simulink model "FullSystem_threshold_fix_attempt"  (R2014a)
settings: Solver=FixedStepDiscrete  StartTime=0.0  StopTime=1.5  FixedStep=1/8000  RelTol=1e-3
undefined symbols (not defined in the file): i
libraries: dspmtrx3 x7, dspsrcs4 x7, commutil2 x1, dspstat3 x1, dspsigops x1, dspbuff3 x1, simulink x1
settings Model: NumberOfSteps=400  Creator=Dolby  LastModifiedBy=100442260
settings DataIOCC: SaveOutput=off  SaveTime=off
settings DebuggingCC: UnderspecifiedInitializationDetection=Classic  StateNameClashWarn=warning

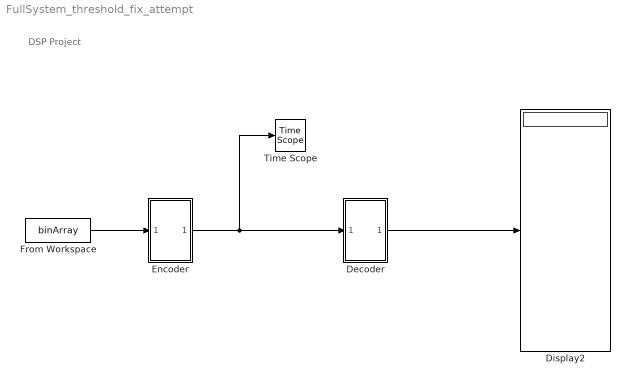
== system FullSystem_threshold_fix_attempt ==
  note: DSP Project
  "Decoder " : Subsystem
  Display2 : Display
  Encoder : Subsystem
  From Workspace : FromWorkspace  VariableName=binArray
  Time Scope : TimeScope  DefaultConfigurationName=spbscopes.TimeScopeBlockCfg
  wires:
  Encoder/1(Out1) -> "Decoder "/1(In1), Time Scope/1
  From Workspace/1 -> Encoder/1(In1)
  "Decoder "/1(Out1) -> Display2/1

== system FullSystem_threshold_fix_attempt/Decoder  ==
  In1 : Inport
  Binary to Decimal : Subsystem
  Delay : Delay  DelayLength=60  InitialCondition=0
  Digitbreak : Subsystem
  "Geortzel Filtering " : Subsystem
  Shift register : Subsystem  TreatAsAtomicUnit=on
  Time Scope1 : TimeScope  DefaultConfigurationName=spbscopes.TimeScopeBlockCfg
  Out1 : Outport
  wires:
  In1/1 -> Digitbreak/1(In1), "Geortzel Filtering "/1(In1)
  "Geortzel Filtering "/1(Out1) -> Binary to Decimal/1(In1)
  Shift register/1(Output) -> Out1/1
  Digitbreak/1(Out2) -> Time Scope1/1, Delay/1, Binary to Decimal/2(In2), "Geortzel Filtering "/2(In2)  "Trigger"
  Binary to Decimal/1(Out2) -> Shift register/1(Input)
  Delay/1 -> Shift register/Trigger

== system FullSystem_threshold_fix_attempt/Encoder ==
  In1 : Inport
  Noise : Subsystem
  Tone Generator : Subsystem
  Out1 : Outport
  wires:
  In1/1 -> Tone Generator/1(In1)
  Tone Generator/1(Out1) -> Noise/1(In1)
  Noise/1(Out1) -> Out1/1

== system FullSystem_threshold_fix_attempt/Decoder /Binary to Decimal ==
  In1 : Inport
  In2 : Inport  Port=2
  Delay : Delay  DelayLength=60  InitialCondition=0
  Triggered Subsystem : Subsystem  TreatAsAtomicUnit=on
  Out2 : Outport
  wires:
  Delay/1 -> Triggered Subsystem/Trigger
  In1/1 -> Triggered Subsystem/1(In1)
  In2/1 -> Delay/1
  Triggered Subsystem/1(Out1) -> Out2/1

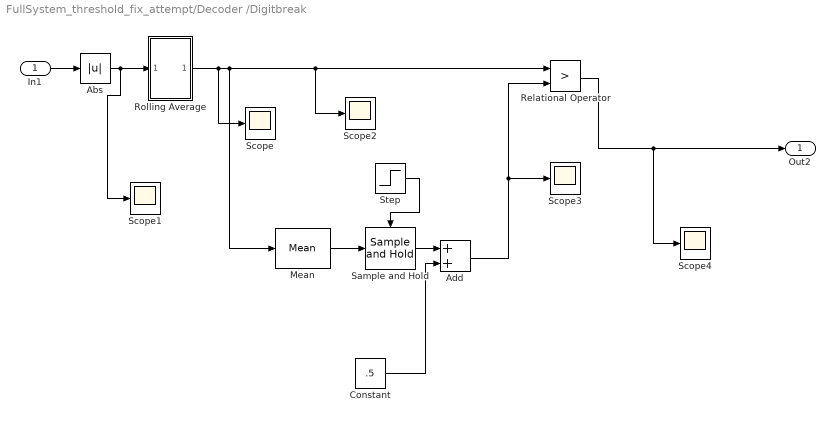
== system FullSystem_threshold_fix_attempt/Decoder /Digitbreak ==
  In1 : Inport
  Abs : Abs
  Add : Sum
  Constant : Constant  Value=.5
  Mean : dspstat3/Mean  run=on  reset_popup=None  InputProcessing=Columns as channels (frame based)  directionMode=Each column  dimension=1  treatSBRowAsCol=on  roiEnable=off  roiType=Rectangles  roiPortion=Entire ROI  roiOutput=Individual statistics for each ROI  roiFlag=off  outputDataTypeStr=Inherit: Same as accumulator  outputLastDataTypeStr=Inherit: Same as accumulator  outputMin=[]  outputMax=[]  roundingMode=Floor  overflowMode=off
  Relational Operator : RelationalOperator  Operator=>  OutDataTypeStr=boolean
  Rolling Average : Subsystem
  Sample and Hold : dspsigops/Sample and Hold  trig=Rising edge  initCond=.5  latchinput=off
  Scope{,1..4} (5 alike) : Scope
      Scope settings: SaveName=ScopeData21
      Scope1 settings: SaveName=ScopeData19
      Scope2 settings: SaveName=ScopeData20
      Scope3 settings: SaveName=ScopeData7
      Scope4 settings: SaveName=ScopeData24
  Step : Step  Time=.05  SampleTime=0
  Out2 : Outport
  wires:
  Abs/1 -> Scope1/1, Rolling Average/1(In1)
  In1/1 -> Abs/1
  Relational Operator/1 -> Scope4/1, Out2/1
  Step/1 -> Sample and Hold/Trigger
  Rolling Average/1(Out1) -> Scope/1, Scope2/1, Relational Operator/1, Mean/1
  Mean/1 -> Sample and Hold/1
  Add/1 -> Scope3/1, Relational Operator/2
  Sample and Hold/1 -> Add/1
  Constant/1 -> Add/2

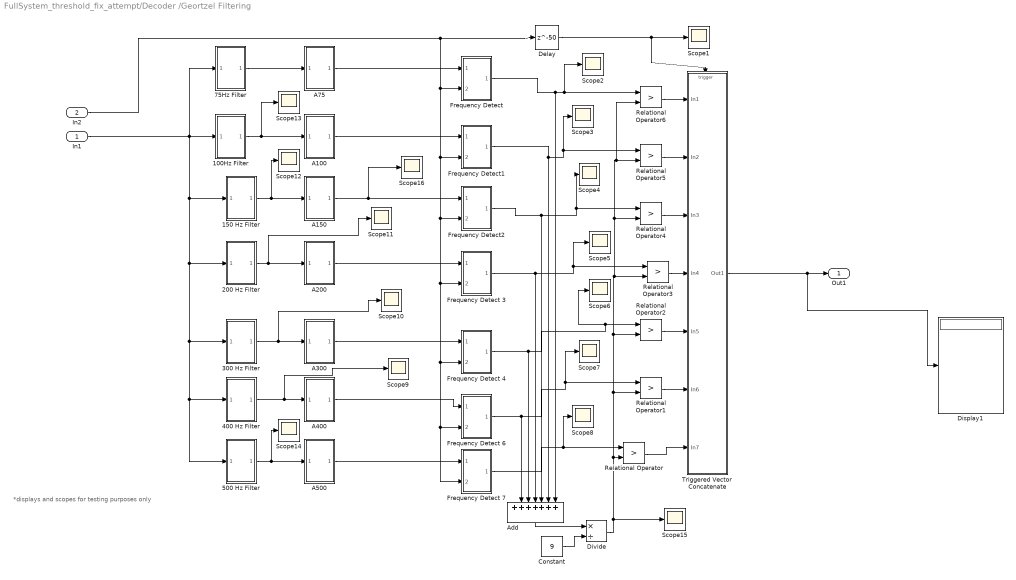
== system FullSystem_threshold_fix_attempt/Decoder /Geortzel Filtering  ==
  note: *displays and scopes for testing purposes only
  In1 : Inport
  In2 : Inport  Port=2
  100Hz Filter : Subsystem
  150 Hz Filter : Subsystem
  200 Hz Filter : Subsystem
  "300 Hz Filter " : Subsystem
  400 Hz Filter : Subsystem
  500 Hz Filter : Subsystem
  75Hz Filter : Subsystem
  A100 : Subsystem
  A150 : Subsystem
  "A200 " : Subsystem
  A300 : Subsystem
  A400 : Subsystem
  A500 : Subsystem
  A75 : Subsystem
  Add : Sum  Inputs=+++++++
  Constant : Constant  Value=9
  Delay : Delay  DelayLength=50  InitialCondition=0
  Display1 : Display
  Divide : Product  Inputs=*/
  Frequency Detect : Subsystem
  "Frequency Detect 3 " : Subsystem
  Frequency Detect 4 : Subsystem
  "Frequency Detect 6 " : Subsystem
  "Frequency Detect 7 " : Subsystem
  "Frequency Detect1 " : Subsystem
  "Frequency Detect2 " : Subsystem
  Relational Operator{,1..6} (7 alike) : RelationalOperator  Operator=>  OutDataTypeStr=boolean
  Scope{1..16} (16 alike) : Scope
      Scope1 settings: TimeRange=0.2  YMin=-2  YMax=2
      Scope10 settings: TimeRange=0.2  YMin=-2  YMax=2  SaveName=ScopeData12
      Scope11 settings: TimeRange=0.2  YMin=-2  YMax=2  SaveName=ScopeData13
      Scope12 settings: TimeRange=0.2  YMin=-2  YMax=2  SaveName=ScopeData14
      Scope13 settings: TimeRange=0.2  YMin=-2  YMax=2  SaveName=ScopeData15
      Scope14 settings: TimeRange=0.2  YMin=-2  YMax=2  SaveName=ScopeData16
      Scope15 settings: TimeRange=0.08000000000000002  YMin=-0.1  YMax=1.3
      Scope16 settings: TimeRange=0.2  YMin=-2  YMax=2  SaveName=ScopeData17
      Scope2 settings: TimeRange=0.2  YMin=-2  YMax=2  SaveName=ScopeData2
      Scope3 settings: TimeRange=0.2  YMin=-2  YMax=2  SaveName=ScopeData4
      Scope4 settings: TimeRange=0.2  YMin=-2  YMax=2  SaveName=ScopeData5
      Scope5 settings: TimeRange=0.2  YMin=-2  YMax=2  SaveName=ScopeData6
      Scope6 settings: TimeRange=0.2  YMin=-2  YMax=2  SaveName=ScopeData8
      Scope7 settings: TimeRange=0.2  YMin=-2  YMax=2  SaveName=ScopeData9
      Scope8 settings: TimeRange=0.2  YMin=-2  YMax=2  SaveName=ScopeData10
      Scope9 settings: TimeRange=0.2  YMin=-2  YMax=2  SaveName=ScopeData11
  Triggered Vector Concatenate : Subsystem
  Out1 : Outport
  wires:
  100Hz Filter/1(Out1) -> Scope13/1, A100/1(In1)
  "300 Hz Filter "/1(Out1) -> Scope10/1, A300/1(In1)
  75Hz Filter/1(Out1) -> A75/1(In1)
  150 Hz Filter/1(Out1) -> Scope12/1, A150/1(In1)
  500 Hz Filter/1(Out1) -> Scope14/1, A500/1(In1)
  A75/1(Out1) -> Frequency Detect/1(In3)
  In1/1 -> 400 Hz Filter/1(In1), 500 Hz Filter/1(In1), "300 Hz Filter "/1(In1), 200 Hz Filter/1(In1), 150 Hz Filter/1(In1), 75Hz Filter/1(In1), 100Hz Filter/1(In1)
  A100/1(Out1) -> "Frequency Detect1 "/1(In3)
  In2/1 -> Frequency Detect/2(In1), "Frequency Detect 7 "/2(In1), "Frequency Detect 6 "/2(In1), Frequency Detect 4/2(In1), "Frequency Detect 3 "/2(In1), "Frequency Detect2 "/2(In1), "Frequency Detect1 "/2(In1), Delay/1
  A150/1(Out1) -> Scope16/1, "Frequency Detect2 "/1(In3)
  "A200 "/1(Out1) -> "Frequency Detect 3 "/1(In3)
  A300/1(Out1) -> Frequency Detect 4/1(In3)
  A400/1(Out1) -> "Frequency Detect 6 "/1(In3)
  A500/1(Out1) -> "Frequency Detect 7 "/1(In3)
  "Frequency Detect2 "/1(Out1) -> Scope4/1, Relational Operator4/1, Add/5
  "Frequency Detect 3 "/1(Out1) -> Add/4, Relational Operator3/1, Scope5/1
  Frequency Detect 4/1(Out1) -> Add/3, Relational Operator2/1, Scope6/1
  "Frequency Detect 6 "/1(Out1) -> Add/2, Relational Operator1/1, Scope7/1
  "Frequency Detect 7 "/1(Out1) -> Relational Operator/1, Scope8/1
  Delay/1 -> Scope1/1, Triggered Vector Concatenate/Trigger
  Triggered Vector Concatenate/1(Out1) -> Out1/1, Display1/1
  200 Hz Filter/1(Out1) -> Scope11/1, "A200 "/1(In1)
  400 Hz Filter/1(Out1) -> Scope9/1, A400/1(In1)
  Relational Operator/1 -> Triggered Vector Concatenate/7(In7)
  Add/1 -> Divide/1
  Constant/1 -> Divide/2
  Relational Operator1/1 -> Triggered Vector Concatenate/6(In6)
  Relational Operator2/1 -> Triggered Vector Concatenate/5(In5)
  Divide/1 -> Scope15/1, Relational Operator6/2, Relational Operator5/2, Relational Operator4/2, Relational Operator3/2, Relational Operator2/2, Relational Operator1/2, Relational Operator/2
  Relational Operator3/1 -> Triggered Vector Concatenate/4(In4)
  Relational Operator4/1 -> Triggered Vector Concatenate/3(In3)
  Relational Operator5/1 -> Triggered Vector Concatenate/2(In2)
  Relational Operator6/1 -> Triggered Vector Concatenate/1(In1)
  Frequency Detect/1(Out1) -> Add/7, Relational Operator6/1, Scope2/1
  "Frequency Detect1 "/1(Out1) -> Add/6, Relational Operator5/1, Scope3/1

== system FullSystem_threshold_fix_attempt/Decoder /Shift register ==
  Input : Inport
  Trigger : TriggerPort  TriggerType=falling  ZeroCross=off
  Delay Line : dspbuff3/Delay Line  siz=11  ic=0  directfeed=on  enable_output=off  hold_output=off  TreatMby1Signals=One channel
  Output : Outport
  wires:
  Input/1 -> Delay Line/1
  Delay Line/1 -> Output/1

== system FullSystem_threshold_fix_attempt/Encoder/Noise ==
  In1 : Inport
  Add : Sum
  Band-Limited White Noise : simulink/Sources/Band-Limited White Noise  Cov=[0.0000005]  Ts=1/8000  seed=[1]
  Scope : Scope
      settings: SaveName=ScopeData22
  Out1 : Outport
  wires:
  In1/1 -> Add/2
  Band-Limited White Noise/1 -> Add/1
  Add/1 -> Scope/1, Out1/1

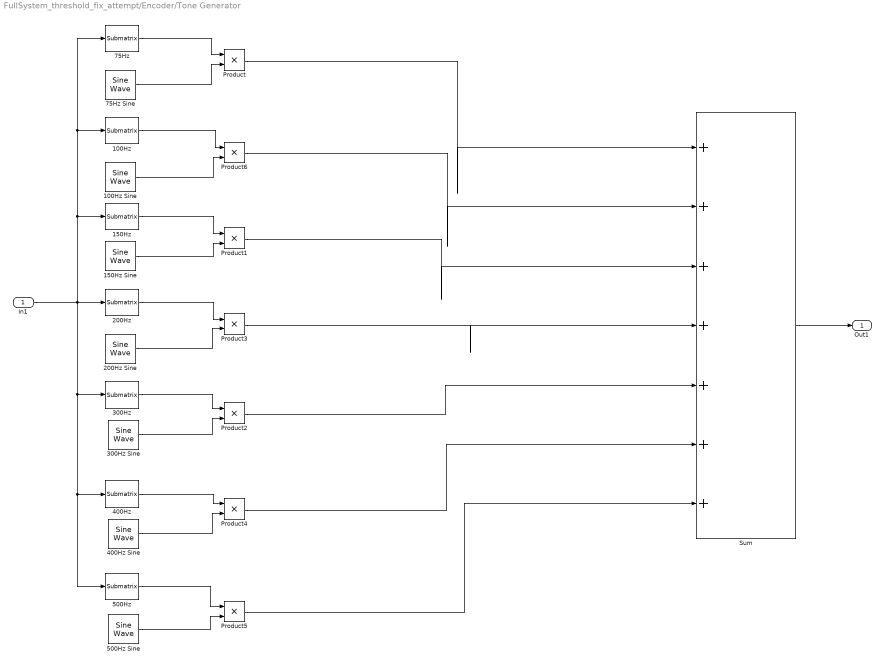
== system FullSystem_threshold_fix_attempt/Encoder/Tone Generator ==
  In1 : Inport
  100Hz : dspmtrx3/Submatrix  RowSpan=One row  RowStartMode=Index  RowStartIndex=2  RowEndMode=Last  RowEndIndex=1  ColSpan=Range of columns  ColStartMode=First  ColStartIndex=1  ColEndMode=Last  ColEndIndex=1
  100Hz Sine : dspsrcs4/Sine Wave  Amplitude=1 + rand()  Frequency=100  Phase=0  SampleMode=Discrete  OutComplex=Real  CompMethod=Trigonometric fcn  TableSize=Speed  SampleTime=1/8000  SamplesPerFrame=1  ResetState=Restart at time zero  dataType=double  wordLen=16  udDataType=sfix(16)  fracBitsMode=Best precision  numFracBits=15  OutDataTypeStr=double  LastOutDataTypeStr=double
  150Hz : dspmtrx3/Submatrix  RowSpan=One row  RowStartMode=Index  RowStartIndex=3  RowEndMode=Last  RowEndIndex=1  ColSpan=Range of columns  ColStartMode=First  ColStartIndex=1  ColEndMode=Last  ColEndIndex=1
  150Hz Sine : dspsrcs4/Sine Wave  Amplitude=1 + rand()  Frequency=150  Phase=0  SampleMode=Discrete  OutComplex=Real  CompMethod=Trigonometric fcn  TableSize=Speed  SampleTime=1/8000  SamplesPerFrame=1  ResetState=Restart at time zero  dataType=double  wordLen=16  udDataType=sfix(16)  fracBitsMode=Best precision  numFracBits=15  OutDataTypeStr=double  LastOutDataTypeStr=double
  200Hz : dspmtrx3/Submatrix  RowSpan=One row  RowStartMode=Index  RowStartIndex=4  RowEndMode=Last  RowEndIndex=1  ColSpan=Range of columns  ColStartMode=First  ColStartIndex=1  ColEndMode=Last  ColEndIndex=1
  200Hz Sine : dspsrcs4/Sine Wave  Amplitude=1 + rand()  Frequency=200  Phase=0  SampleMode=Discrete  OutComplex=Real  CompMethod=Trigonometric fcn  TableSize=Speed  SampleTime=1/8000  SamplesPerFrame=1  ResetState=Restart at time zero  dataType=double  wordLen=16  udDataType=sfix(16)  fracBitsMode=Best precision  numFracBits=15  OutDataTypeStr=double  LastOutDataTypeStr=double
  300Hz : dspmtrx3/Submatrix  RowSpan=One row  RowStartMode=Index  RowStartIndex=5  RowEndMode=Last  RowEndIndex=1  ColSpan=Range of columns  ColStartMode=First  ColStartIndex=1  ColEndMode=Last  ColEndIndex=1
  300Hz Sine : dspsrcs4/Sine Wave  Amplitude=1 + rand()  Frequency=300  Phase=0  SampleMode=Discrete  OutComplex=Real  CompMethod=Trigonometric fcn  TableSize=Speed  SampleTime=1/8000  SamplesPerFrame=1  ResetState=Restart at time zero  dataType=double  wordLen=16  udDataType=sfix(16)  fracBitsMode=Best precision  numFracBits=15  OutDataTypeStr=double  LastOutDataTypeStr=double
  400Hz : dspmtrx3/Submatrix  RowSpan=One row  RowStartMode=Index  RowStartIndex=6  RowEndMode=Last  RowEndIndex=1  ColSpan=Range of columns  ColStartMode=First  ColStartIndex=1  ColEndMode=Last  ColEndIndex=1
  400Hz Sine : dspsrcs4/Sine Wave  Amplitude=1 + rand()  Frequency=400  Phase=0  SampleMode=Discrete  OutComplex=Real  CompMethod=Trigonometric fcn  TableSize=Speed  SampleTime=1/8000  SamplesPerFrame=1  ResetState=Restart at time zero  dataType=double  wordLen=16  udDataType=sfix(16)  fracBitsMode=Best precision  numFracBits=15  OutDataTypeStr=double  LastOutDataTypeStr=double
  500Hz : dspmtrx3/Submatrix  RowSpan=One row  RowStartMode=Last  RowStartIndex=1  RowEndMode=Last  RowEndIndex=1  ColSpan=Range of columns  ColStartMode=First  ColStartIndex=1  ColEndMode=Last  ColEndIndex=1
  500Hz Sine : dspsrcs4/Sine Wave  Amplitude=1 + rand()  Frequency=500  Phase=0  SampleMode=Discrete  OutComplex=Real  CompMethod=Trigonometric fcn  TableSize=Speed  SampleTime=1/8000  SamplesPerFrame=1  ResetState=Restart at time zero  dataType=double  wordLen=16  udDataType=sfix(16)  fracBitsMode=Best precision  numFracBits=15  OutDataTypeStr=double  LastOutDataTypeStr=double
  75Hz : dspmtrx3/Submatrix  RowSpan=One row  RowStartMode=First  RowStartIndex=1  RowEndMode=Last  RowEndIndex=1  ColSpan=Range of columns  ColStartMode=First  ColStartIndex=1  ColEndMode=Last  ColEndIndex=1
  75Hz Sine : dspsrcs4/Sine Wave  Amplitude=1 + rand()  Frequency=75  Phase=0  SampleMode=Discrete  OutComplex=Real  CompMethod=Trigonometric fcn  TableSize=Speed  SampleTime=1/8000  SamplesPerFrame=1  ResetState=Restart at time zero  dataType=double  wordLen=16  udDataType=sfix(16)  fracBitsMode=Best precision  numFracBits=15  OutDataTypeStr=double  LastOutDataTypeStr=double
  Product{,1..6} (7 alike) : Product
  Sum : Sum  Inputs=|+++++++
  Out1 : Outport
  wires:
  150Hz/1 -> Product1/1
  150Hz Sine/1 -> Product1/2
  200Hz/1 -> Product3/1
  100Hz Sine/1 -> Product6/2
  100Hz/1 -> Product6/1
  300Hz/1 -> Product2/1
  75Hz/1 -> Product/1
  400Hz/1 -> Product4/1
  500Hz/1 -> Product5/1
  Product/1 -> Sum/1
  Product6/1 -> Sum/2
  Product1/1 -> Sum/3
  Product3/1 -> Sum/4
  Product2/1 -> Sum/5
  Product4/1 -> Sum/6
  Product5/1 -> Sum/7
  Sum/1 -> Out1/1
  75Hz Sine/1 -> Product/2
  200Hz Sine/1 -> Product3/2
  300Hz Sine/1 -> Product2/2
  400Hz Sine/1 -> Product4/2
  500Hz Sine/1 -> Product5/2
  In1/1 -> 200Hz/1, 150Hz/1, 100Hz/1, 75Hz/1, 300Hz/1, 400Hz/1, 500Hz/1

== system FullSystem_threshold_fix_attempt/Decoder /Binary to Decimal/Triggered Subsystem ==
  In1 : Inport
  Trigger : TriggerPort  TriggerType=falling
  A1 : Constant  Value=[0; 1; 2; 3; 4; 5; 6; 7; 8; 9]
  A11 : Constant  Value=[84; 44; 42; 41; 52; 50; 49; 76; 74; 73]
  Bit to Integer Converter : commutil2/Bit to Integer Converter  nbits=7  bitOrder=MSB first  signedOutputValues=Unsigned  outDtype=Inherit via internal rule  outDtypeSigned=Inherit via internal rule
  Display : Display
  Matrix Sum : Sum  Inputs=+  OutDataTypeStr=double
  Matrix Multiply : Product
  Relational Operator : RelationalOperator  Operator===  OutDataTypeStr=boolean
  Out1 : Outport
  wires:
  A11/1 -> Relational Operator/2
  Matrix Sum/1 -> Out1/1
  In1/1 -> Bit to Integer Converter/1
  Bit to Integer Converter/1 -> Display/1, Relational Operator/1
  Relational Operator/1 -> Matrix Multiply/1
  A1/1 -> Matrix Multiply/2
  Matrix Multiply/1 -> Matrix Sum/1

== system FullSystem_threshold_fix_attempt/Decoder /Digitbreak/Rolling Average ==
  In1 : Inport
  Subsystem : Subsystem
  Out1 : Outport
  wires:
  In1/1 -> Subsystem/1(In1)
  Subsystem/1(Out1) -> Out1/1

== system FullSystem_threshold_fix_attempt/Decoder /Geortzel Filtering /100Hz Filter ==
  In1 : Inport
  Add3 : Sum
  Add4 : Sum  Inputs=-+
  Add5 : Sum
  Gain3 : Gain
  Gain4 : Gain  Gain=-cos(2*pi*5/400)-(sin(2*pi*5/400)*i)
  Gain5 : Gain  Gain=2*cos(2*pi*5/400)
  Unit Delay : UnitDelay  SampleTime=-1
  Unit Delay1 : UnitDelay  SampleTime=-1
  Out1 : Outport
  wires:
  In1/1 -> Add3/1
  Add4/1 -> Add3/2
  Gain3/1 -> Add4/1
  Add3/1 -> Unit Delay/1, Add5/1
  Add5/1 -> Out1/1
  Gain5/1 -> Add4/2
  Gain4/1 -> Add5/2
  Unit Delay1/1 -> Gain3/1
  Unit Delay/1 -> Gain4/1, Unit Delay1/1, Gain5/1

== system FullSystem_threshold_fix_attempt/Decoder /Geortzel Filtering /150 Hz Filter ==
  In1 : Inport
  Add6 : Sum
  Add7 : Sum  Inputs=-+
  Add8 : Sum
  Gain6 : Gain
  Gain7 : Gain  Gain=-cos(2*pi*7.5/400)-(sin(2*pi*7.5/400)*i)
  Gain8 : Gain  Gain=2*cos(2*pi*7.5/400)
  Unit Delay : UnitDelay  SampleTime=-1
  Unit Delay1 : UnitDelay  SampleTime=-1
  Out1 : Outport
  wires:
  In1/1 -> Add6/1
  Gain7/1 -> Add8/2
  Add8/1 -> Out1/1
  Gain8/1 -> Add7/2
  Add7/1 -> Add6/2
  Gain6/1 -> Add7/1
  Add6/1 -> Unit Delay/1, Add8/1
  Unit Delay1/1 -> Gain6/1
  Unit Delay/1 -> Gain7/1, Unit Delay1/1, Gain8/1

== system FullSystem_threshold_fix_attempt/Decoder /Geortzel Filtering /200 Hz Filter ==
  In1 : Inport
  Add10 : Sum  Inputs=-+
  Add11 : Sum
  Add9 : Sum
  Gain10 : Gain  Gain=-cos(2*pi*10/400)-(sin(2*pi*10/400)*i)
  Gain11 : Gain  Gain=2*cos(2*pi*10/400)
  Gain9 : Gain
  Unit Delay : UnitDelay  SampleTime=-1
  Unit Delay1 : UnitDelay  SampleTime=-1
  Out1 : Outport
  wires:
  Gain10/1 -> Add11/2
  Unit Delay1/1 -> Unit Delay/1, Gain10/1, Gain11/1
  Gain9/1 -> Add10/1
  Add10/1 -> Add9/2
  Unit Delay/1 -> Gain9/1
  Add11/1 -> Out1/1
  Add9/1 -> Unit Delay1/1, Add11/1
  Gain11/1 -> Add10/2
  In1/1 -> Add9/1

== system FullSystem_threshold_fix_attempt/Decoder /Geortzel Filtering /300 Hz Filter  ==
  In1 : Inport
  Add12 : Sum
  Add13 : Sum  Inputs=-+
  Add14 : Sum
  Gain12 : Gain
  Gain13 : Gain  Gain=-cos(2*pi*15/400)-(sin(2*pi*15/400)*i)
  Gain14 : Gain  Gain=2*cos(2*pi*15/400)
  Unit Delay : UnitDelay  SampleTime=-1
  Unit Delay1 : UnitDelay  SampleTime=-1
  Out1 : Outport
  wires:
  Add14/1 -> Out1/1
  Add12/1 -> Unit Delay1/1, Add14/1
  Gain12/1 -> Add13/1
  Unit Delay1/1 -> Unit Delay/1, Gain13/1, Gain14/1
  Add13/1 -> Add12/2
  Gain13/1 -> Add14/2
  Unit Delay/1 -> Gain12/1
  Gain14/1 -> Add13/2
  In1/1 -> Add12/1

== system FullSystem_threshold_fix_attempt/Decoder /Geortzel Filtering /400 Hz Filter ==
  In1 : Inport
  Add18 : Sum
  Add19 : Sum  Inputs=-+
  Add20 : Sum
  Gain18 : Gain
  Gain19 : Gain  Gain=-cos(2*pi*21/400)-(sin(2*pi*20/400)*i)  SampleTime=1/8000
  Gain20 : Gain  Gain=2*cos(2*pi*20/400)  SampleTime=1/8000
  Unit Delay : UnitDelay  SampleTime=-1
  Unit Delay1 : UnitDelay  SampleTime=-1
  Out1 : Outport
  wires:
  Unit Delay1/1 -> Unit Delay/1, Gain19/1, Gain20/1
  Add19/1 -> Add18/2
  Add18/1 -> Unit Delay1/1, Add20/1
  Gain18/1 -> Add19/1
  Unit Delay/1 -> Gain18/1
  Add20/1 -> Out1/1
  Gain19/1 -> Add20/2
  Gain20/1 -> Add19/2
  In1/1 -> Add18/1

== system FullSystem_threshold_fix_attempt/Decoder /Geortzel Filtering /500 Hz Filter ==
  In1 : Inport
  Add18 : Sum
  Add19 : Sum  Inputs=-+
  Add20 : Sum
  Gain18 : Gain
  Gain19 : Gain  Gain=-cos(2*pi*25/400)-(sin(2*pi*25/400)*i)
  Gain20 : Gain  Gain=2*cos(2*pi*25/400)
  Unit Delay : UnitDelay  SampleTime=-1
  Unit Delay1 : UnitDelay  SampleTime=-1
  Out1 : Outport
  wires:
  Unit Delay1/1 -> Unit Delay/1, Gain19/1, Gain20/1
  Add19/1 -> Add18/2
  Add18/1 -> Unit Delay1/1, Add20/1
  Gain18/1 -> Add19/1
  Unit Delay/1 -> Gain18/1
  Add20/1 -> Out1/1
  Gain19/1 -> Add20/2
  Gain20/1 -> Add19/2
  In1/1 -> Add18/1

== system FullSystem_threshold_fix_attempt/Decoder /Geortzel Filtering /75Hz Filter ==
  In1 : Inport
  Add : Sum  InputSameDT=on
  Add1 : Sum  Inputs=-+
  Add2 : Sum  InputSameDT=on
  Gain : Gain
  Gain1 : Gain  Gain=-cos(2*pi*3.75/400)-(sin(2*pi*3.75/400)*i)
  Gain2 : Gain  Gain=2*cos(2*pi*3.75/400)
  Unit Delay : UnitDelay  SampleTime=-1
  Unit Delay1 : UnitDelay  SampleTime=-1
  Out1 : Outport
  wires:
  In1/1 -> Add/1
  Add2/1 -> Out1/1
  Gain/1 -> Add1/1
  Gain2/1 -> Add1/2
  Gain1/1 -> Add2/2
  Add1/1 -> Add/2
  Add/1 -> Unit Delay/1, Add2/1
  Unit Delay1/1 -> Gain/1
  Unit Delay/1 -> Unit Delay1/1, Gain1/1, Gain2/1

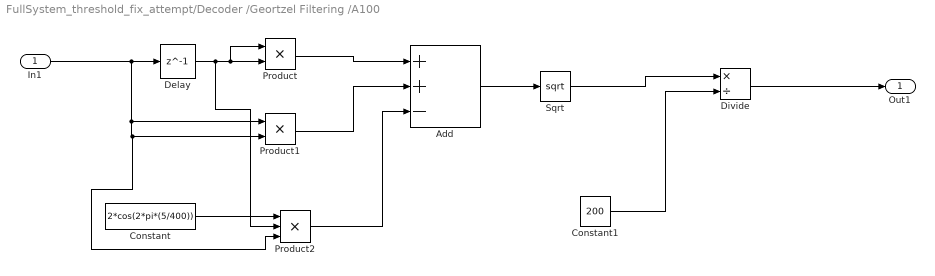
== system FullSystem_threshold_fix_attempt/Decoder /Geortzel Filtering /A100 ==
  In1 : Inport
  Add : Sum  Inputs=++-
  Constant : Constant  Value=2*cos(2*pi*(5/400))
  Constant1 : Constant  Value=200
  Delay : Delay  DelayLength=1  InitialCondition=0
  Divide : Product  Inputs=*/
  Product : Product
  Product1 : Product
  Product2 : Product  Inputs=3
  Sqrt : Sqrt  SaturateOnIntegerOverflow=on
  Out1 : Outport
  wires:
  In1/1 -> Delay/1, Product2/3, Product1/2, Product1/1
  Delay/1 -> Product2/2, Product/1, Product/2
  Product/1 -> Add/1
  Product1/1 -> Add/2
  Constant/1 -> Product2/1
  Add/1 -> Sqrt/1
  Product2/1 -> Add/3
  Sqrt/1 -> Divide/1
  Constant1/1 -> Divide/2
  Divide/1 -> Out1/1

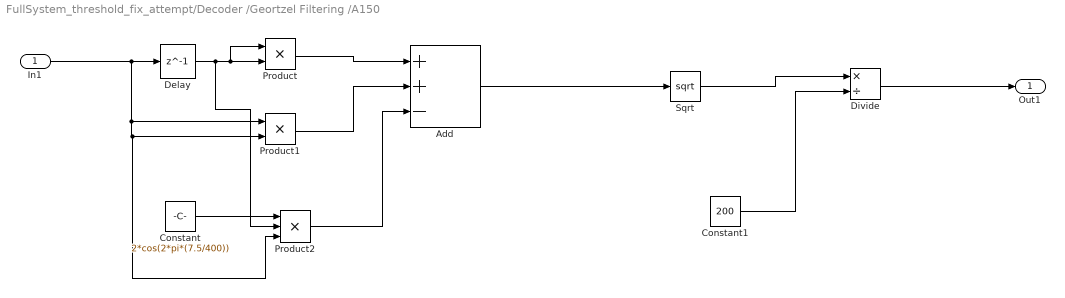
== system FullSystem_threshold_fix_attempt/Decoder /Geortzel Filtering /A150 ==
  In1 : Inport
  Add : Sum  Inputs=++-
  Constant : Constant  Value=2*cos(2*pi*(7.5/400))
  Constant1 : Constant  Value=200
  Delay : Delay  DelayLength=1  InitialCondition=0
  Divide : Product  Inputs=*/
  Product : Product
  Product1 : Product
  Product2 : Product  Inputs=3
  Sqrt : Sqrt  SaturateOnIntegerOverflow=on
  Out1 : Outport
  wires:
  In1/1 -> Delay/1, Product2/3, Product1/2, Product1/1
  Delay/1 -> Product2/2, Product/1, Product/2
  Product/1 -> Add/1
  Product1/1 -> Add/2
  Constant/1 -> Product2/1
  Add/1 -> Sqrt/1
  Product2/1 -> Add/3
  Sqrt/1 -> Divide/1
  Constant1/1 -> Divide/2
  Divide/1 -> Out1/1

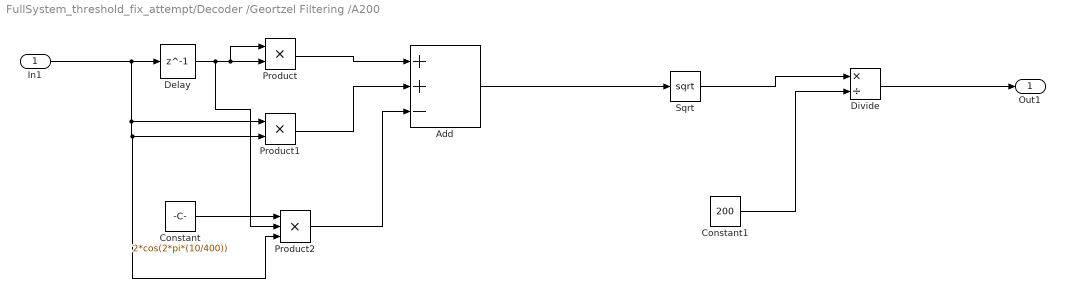
== system FullSystem_threshold_fix_attempt/Decoder /Geortzel Filtering /A200  ==
  In1 : Inport
  Add : Sum  Inputs=++-
  Constant : Constant  Value=2*cos(2*pi*(10/400))
  Constant1 : Constant  Value=200
  Delay : Delay  DelayLength=1  InitialCondition=0
  Divide : Product  Inputs=*/
  Product : Product
  Product1 : Product
  Product2 : Product  Inputs=3
  Sqrt : Sqrt  SaturateOnIntegerOverflow=on
  Out1 : Outport
  wires:
  In1/1 -> Delay/1, Product2/3, Product1/2, Product1/1
  Delay/1 -> Product2/2, Product/1, Product/2
  Product/1 -> Add/1
  Product1/1 -> Add/2
  Constant/1 -> Product2/1
  Add/1 -> Sqrt/1
  Product2/1 -> Add/3
  Sqrt/1 -> Divide/1
  Constant1/1 -> Divide/2
  Divide/1 -> Out1/1

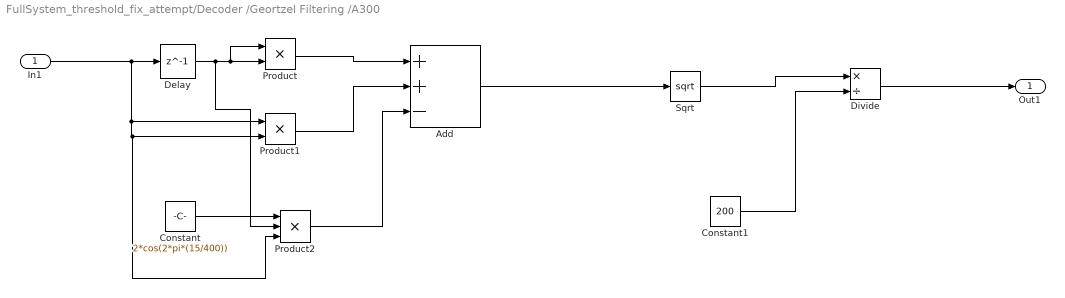
== system FullSystem_threshold_fix_attempt/Decoder /Geortzel Filtering /A300 ==
  In1 : Inport
  Add : Sum  Inputs=++-
  Constant : Constant  Value=2*cos(2*pi*(15/400))
  Constant1 : Constant  Value=200
  Delay : Delay  DelayLength=1  InitialCondition=0
  Divide : Product  Inputs=*/
  Product : Product
  Product1 : Product
  Product2 : Product  Inputs=3
  Sqrt : Sqrt  SaturateOnIntegerOverflow=on
  Out1 : Outport
  wires:
  In1/1 -> Delay/1, Product2/3, Product1/2, Product1/1
  Delay/1 -> Product2/2, Product/1, Product/2
  Product/1 -> Add/1
  Product1/1 -> Add/2
  Constant/1 -> Product2/1
  Add/1 -> Sqrt/1
  Product2/1 -> Add/3
  Sqrt/1 -> Divide/1
  Constant1/1 -> Divide/2
  Divide/1 -> Out1/1

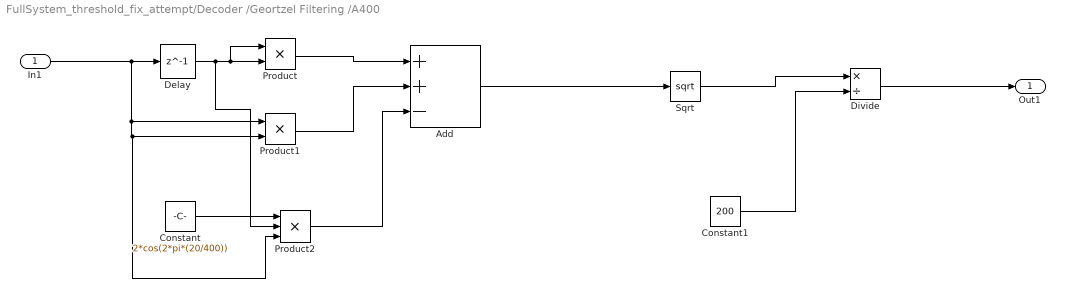
== system FullSystem_threshold_fix_attempt/Decoder /Geortzel Filtering /A400 ==
  In1 : Inport
  Add : Sum  Inputs=++-
  Constant : Constant  Value=2*cos(2*pi*(20/400))
  Constant1 : Constant  Value=200
  Delay : Delay  DelayLength=1  InitialCondition=0
  Divide : Product  Inputs=*/
  Product : Product
  Product1 : Product
  Product2 : Product  Inputs=3
  Sqrt : Sqrt  SaturateOnIntegerOverflow=on
  Out1 : Outport
  wires:
  In1/1 -> Delay/1, Product2/3, Product1/2, Product1/1
  Delay/1 -> Product2/2, Product/1, Product/2
  Product/1 -> Add/1
  Product1/1 -> Add/2
  Constant/1 -> Product2/1
  Add/1 -> Sqrt/1
  Product2/1 -> Add/3
  Sqrt/1 -> Divide/1
  Constant1/1 -> Divide/2
  Divide/1 -> Out1/1

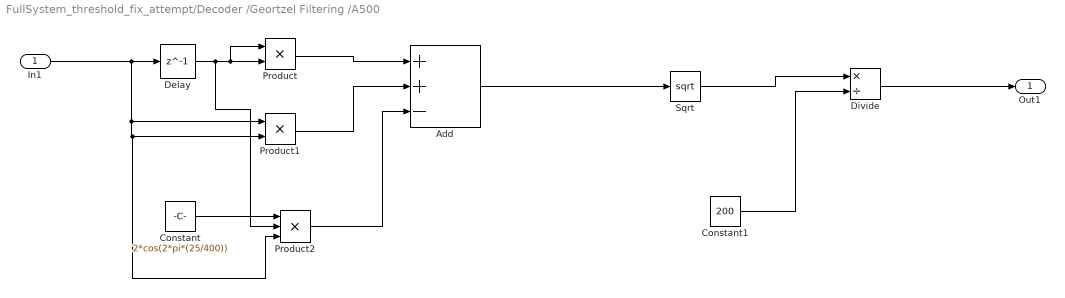
== system FullSystem_threshold_fix_attempt/Decoder /Geortzel Filtering /A500 ==
  In1 : Inport
  Add : Sum  Inputs=++-
  Constant : Constant  Value=2*cos(2*pi*(25/400))
  Constant1 : Constant  Value=200
  Delay : Delay  DelayLength=1  InitialCondition=0
  Divide : Product  Inputs=*/
  Product : Product
  Product1 : Product
  Product2 : Product  Inputs=3
  Sqrt : Sqrt  SaturateOnIntegerOverflow=on
  Out1 : Outport
  wires:
  In1/1 -> Delay/1, Product2/3, Product1/2, Product1/1
  Delay/1 -> Product2/2, Product/1, Product/2
  Product/1 -> Add/1
  Product1/1 -> Add/2
  Constant/1 -> Product2/1
  Add/1 -> Sqrt/1
  Product2/1 -> Add/3
  Sqrt/1 -> Divide/1
  Constant1/1 -> Divide/2
  Divide/1 -> Out1/1

== system FullSystem_threshold_fix_attempt/Decoder /Geortzel Filtering /A75 ==
  In1 : Inport
  Add : Sum  Inputs=++-
  Constant : Constant  Value=2*cos(2*pi*(3.75/400))
  Constant1 : Constant  Value=200
  Delay : Delay  DelayLength=1  InitialCondition=0
  Divide : Product  Inputs=*/
  Product : Product
  Product1 : Product
  Product2 : Product  Inputs=3
  Sqrt : Sqrt  SaturateOnIntegerOverflow=on
  Out1 : Outport
  wires:
  In1/1 -> Delay/1, Product2/3, Product1/2, Product1/1
  Delay/1 -> Product2/2, Product/1, Product/2
  Product/1 -> Add/1
  Product1/1 -> Add/2
  Constant/1 -> Product2/1
  Add/1 -> Sqrt/1
  Product2/1 -> Add/3
  Sqrt/1 -> Divide/1
  Constant1/1 -> Divide/2
  Divide/1 -> Out1/1

== system FullSystem_threshold_fix_attempt/Decoder /Geortzel Filtering /Frequency Detect ==
  In3 : Inport
  In1 : Inport  Port=2
  Gain : Gain  Gain=1.75
  Scope3 : Scope
      settings: TimeRange=0.2  YMin=-2  YMax=2  SaveName=ScopeData3
  Subtract6 : Sum  Inputs=+-
  Triggered Subsystem : Subsystem  TreatAsAtomicUnit=on
  Triggered Subsystem1 : Subsystem  TreatAsAtomicUnit=on
  Out1 : Outport
  wires:
  Subtract6/1 -> Gain/1
  Triggered Subsystem/1(Out1) -> Subtract6/2
  Triggered Subsystem1/1(Out1) -> Subtract6/1
  In3/1 -> Scope3/1, Triggered Subsystem/1(In1), Triggered Subsystem1/1(In1)
  In1/1 -> Triggered Subsystem1/Trigger, Triggered Subsystem/Trigger
  Gain/1 -> Out1/1

== system FullSystem_threshold_fix_attempt/Decoder /Geortzel Filtering /Frequency Detect 3  ==
  In3 : Inport
  In1 : Inport  Port=2
  Scope3 : Scope
      settings: TimeRange=0.2  YMin=0  YMax=1  SaveName=ScopeData3
  Subtract6 : Sum  Inputs=+-
  Triggered Subsystem : Subsystem  TreatAsAtomicUnit=on
  Triggered Subsystem1 : Subsystem  TreatAsAtomicUnit=on
  Out1 : Outport
  wires:
  Subtract6/1 -> Out1/1
  Triggered Subsystem/1(Out1) -> Subtract6/2
  Triggered Subsystem1/1(Out1) -> Subtract6/1
  In3/1 -> Scope3/1, Triggered Subsystem/1(In1), Triggered Subsystem1/1(In1)
  In1/1 -> Triggered Subsystem1/Trigger, Triggered Subsystem/Trigger

== system FullSystem_threshold_fix_attempt/Decoder /Geortzel Filtering /Frequency Detect 4 ==
  In3 : Inport
  In1 : Inport  Port=2
  Scope3 : Scope
      settings: TimeRange=0.2  YMin=0  YMax=1  SaveName=ScopeData3
  Subtract6 : Sum  Inputs=+-
  Triggered Subsystem : Subsystem  TreatAsAtomicUnit=on
  Triggered Subsystem1 : Subsystem  TreatAsAtomicUnit=on
  Out1 : Outport
  wires:
  Subtract6/1 -> Out1/1
  Triggered Subsystem/1(Out1) -> Subtract6/2
  Triggered Subsystem1/1(Out1) -> Subtract6/1
  In3/1 -> Scope3/1, Triggered Subsystem/1(In1), Triggered Subsystem1/1(In1)
  In1/1 -> Triggered Subsystem1/Trigger, Triggered Subsystem/Trigger

== system FullSystem_threshold_fix_attempt/Decoder /Geortzel Filtering /Frequency Detect 6  ==
  In3 : Inport
  In1 : Inport  Port=2
  Scope3 : Scope
      settings: TimeRange=0.2  YMin=0  YMax=1  SaveName=ScopeData3
  Subtract6 : Sum  Inputs=+-
  Triggered Subsystem : Subsystem  TreatAsAtomicUnit=on
  Triggered Subsystem1 : Subsystem  TreatAsAtomicUnit=on
  Out1 : Outport
  wires:
  Subtract6/1 -> Out1/1
  Triggered Subsystem/1(Out1) -> Subtract6/2
  Triggered Subsystem1/1(Out1) -> Subtract6/1
  In3/1 -> Scope3/1, Triggered Subsystem/1(In1), Triggered Subsystem1/1(In1)
  In1/1 -> Triggered Subsystem1/Trigger, Triggered Subsystem/Trigger

== system FullSystem_threshold_fix_attempt/Decoder /Geortzel Filtering /Frequency Detect 7  ==
  In3 : Inport
  In1 : Inport  Port=2
  Scope3 : Scope
      settings: TimeRange=0.2  YMin=0  YMax=1  SaveName=ScopeData3
  Subtract6 : Sum  Inputs=+-
  Triggered Subsystem : Subsystem  TreatAsAtomicUnit=on
  Triggered Subsystem1 : Subsystem  TreatAsAtomicUnit=on
  Out1 : Outport
  wires:
  Subtract6/1 -> Out1/1
  Triggered Subsystem/1(Out1) -> Subtract6/2
  Triggered Subsystem1/1(Out1) -> Subtract6/1
  In3/1 -> Scope3/1, Triggered Subsystem/1(In1), Triggered Subsystem1/1(In1)
  In1/1 -> Triggered Subsystem1/Trigger, Triggered Subsystem/Trigger

== system FullSystem_threshold_fix_attempt/Decoder /Geortzel Filtering /Frequency Detect1  ==
  In3 : Inport
  In1 : Inport  Port=2
  Scope3 : Scope
      settings: TimeRange=0.2  YMin=0  YMax=1  SaveName=ScopeData3
  Subtract6 : Sum  Inputs=+-
  Triggered Subsystem : Subsystem  TreatAsAtomicUnit=on
  Triggered Subsystem1 : Subsystem  TreatAsAtomicUnit=on
  Out1 : Outport
  wires:
  Subtract6/1 -> Out1/1
  Triggered Subsystem/1(Out1) -> Subtract6/2
  Triggered Subsystem1/1(Out1) -> Subtract6/1
  In3/1 -> Scope3/1, Triggered Subsystem/1(In1), Triggered Subsystem1/1(In1)
  In1/1 -> Triggered Subsystem1/Trigger, Triggered Subsystem/Trigger

== system FullSystem_threshold_fix_attempt/Decoder /Geortzel Filtering /Frequency Detect2  ==
  In3 : Inport
  In1 : Inport  Port=2
  Scope3 : Scope
      settings: TimeRange=0.2  YMin=0  YMax=1  SaveName=ScopeData3
  Subtract6 : Sum  Inputs=+-
  Triggered Subsystem : Subsystem  TreatAsAtomicUnit=on
  Triggered Subsystem1 : Subsystem  TreatAsAtomicUnit=on
  Out1 : Outport
  wires:
  Subtract6/1 -> Out1/1
  Triggered Subsystem/1(Out1) -> Subtract6/2
  Triggered Subsystem1/1(Out1) -> Subtract6/1
  In3/1 -> Scope3/1, Triggered Subsystem/1(In1), Triggered Subsystem1/1(In1)
  In1/1 -> Triggered Subsystem1/Trigger, Triggered Subsystem/Trigger

== system FullSystem_threshold_fix_attempt/Decoder /Geortzel Filtering /Triggered Vector Concatenate ==
  In1 : Inport
  In2 : Inport  Port=2
  In3 : Inport  Port=3
  In4 : Inport  Port=4
  In5 : Inport  Port=5
  In6 : Inport  Port=6
  In7 : Inport  Port=7
  Trigger : TriggerPort  TriggerType=falling  ShowOutputPort=on
  Vector Concatenate : Concatenate  NumInputs=7
  Out1 : Outport
  wires:
  In4/1 -> Vector Concatenate/4
  In2/1 -> Vector Concatenate/2
  In6/1 -> Vector Concatenate/6
  In3/1 -> Vector Concatenate/3
  In5/1 -> Vector Concatenate/5
  Vector Concatenate/1 -> Out1/1
  In1/1 -> Vector Concatenate/1
  In7/1 -> Vector Concatenate/7

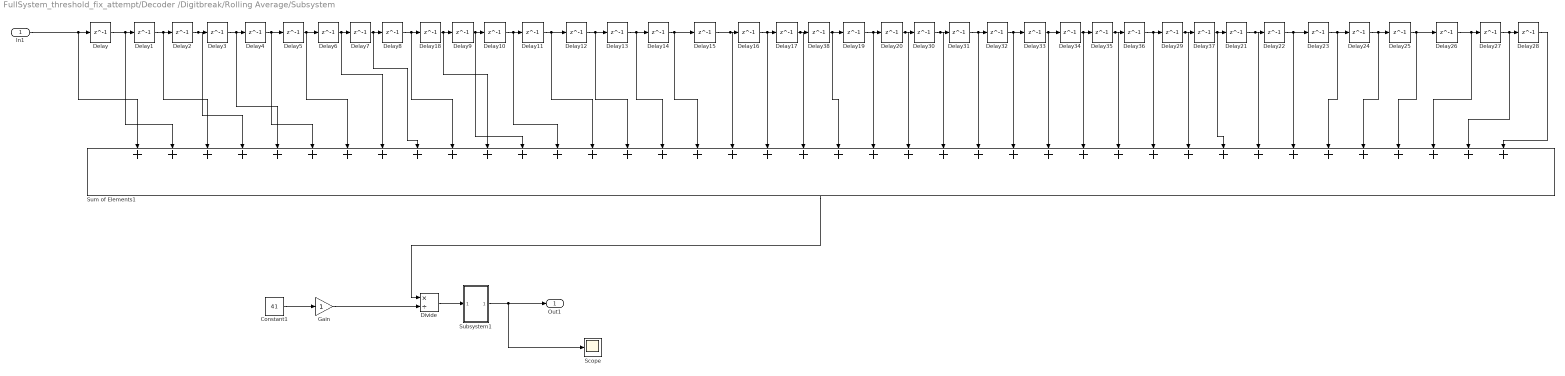
== system FullSystem_threshold_fix_attempt/Decoder /Digitbreak/Rolling Average/Subsystem ==
  In1 : Inport
  Constant1 : Constant  Value=41
  Delay{,1..38} (39 alike) : Delay  DelayLength=1  InitialCondition=0
  Divide : Product  Inputs=*/
  Gain : Gain
  Scope : Scope
      settings: SaveName=ScopeData18
  Subsystem1 : Subsystem
  Sum of Elements1 : Sum  Inputs=++++++++++++++++++++++++++++++++++++++++
  Out1 : Outport
  wires:
  In1/1 -> Sum of Elements1/1, Delay/1
  Delay2/1 -> Sum of Elements1/4, Delay3/1
  Delay5/1 -> Delay6/1, Sum of Elements1/7
  Delay6/1 -> Delay7/1, Sum of Elements1/8
  Delay7/1 -> Sum of Elements1/9, Delay8/1
  Sum of Elements1/1 -> Divide/1
  Delay4/1 -> Delay5/1, Sum of Elements1/6
  Gain/1 -> Divide/2
  Delay3/1 -> Delay4/1, Sum of Elements1/5
  Delay1/1 -> Sum of Elements1/3, Delay2/1
  Constant1/1 -> Gain/1
  Delay/1 -> Sum of Elements1/2, Delay1/1
  Delay8/1 -> Delay18/1, Sum of Elements1/10
  Delay11/1 -> Sum of Elements1/14, Delay12/1
  Delay14/1 -> Sum of Elements1/17, Delay15/1
  Delay15/1 -> Sum of Elements1/18, Delay16/1
  Delay16/1 -> Sum of Elements1/19, Delay17/1
  Delay17/1 -> Sum of Elements1/20, Delay38/1
  Delay13/1 -> Sum of Elements1/16, Delay14/1
  Delay12/1 -> Sum of Elements1/15, Delay13/1
  Delay10/1 -> Sum of Elements1/13, Delay11/1
  Delay9/1 -> Sum of Elements1/12, Delay10/1
  Delay18/1 -> Sum of Elements1/11, Delay9/1
  Delay30/1 -> Sum of Elements1/24, Delay31/1
  Delay33/1 -> Sum of Elements1/27, Delay34/1
  Delay34/1 -> Sum of Elements1/28, Delay35/1
  Delay35/1 -> Sum of Elements1/29, Delay36/1
  Delay32/1 -> Sum of Elements1/26, Delay33/1
  Delay31/1 -> Sum of Elements1/25, Delay32/1
  Delay20/1 -> Sum of Elements1/23, Delay30/1
  Delay36/1 -> Sum of Elements1/30, Delay29/1
  Delay22/1 -> Sum of Elements1/34, Delay23/1
  Delay25/1 -> Sum of Elements1/37, Delay26/1
  Delay26/1 -> Sum of Elements1/38, Delay27/1
  Delay27/1 -> Sum of Elements1/39, Delay28/1
  Delay28/1 -> Sum of Elements1/40
  Delay24/1 -> Sum of Elements1/36, Delay25/1
  Delay23/1 -> Sum of Elements1/35, Delay24/1
  Delay21/1 -> Sum of Elements1/33, Delay22/1
  Delay37/1 -> Sum of Elements1/32, Delay21/1
  Delay29/1 -> Sum of Elements1/31, Delay37/1
  Delay38/1 -> Delay19/1, Sum of Elements1/21
  Delay19/1 -> Sum of Elements1/22, Delay20/1
  Divide/1 -> Subsystem1/1(In1)
  Subsystem1/1(Out1) -> Scope/1, Out1/1

== system FullSystem_threshold_fix_attempt/Decoder /Geortzel Filtering /Frequency Detect/Triggered Subsystem ==
  In1 : Inport
  Trigger : TriggerPort
  Out1 : Outport
  wires:
  In1/1 -> Out1/1

== system FullSystem_threshold_fix_attempt/Decoder /Geortzel Filtering /Frequency Detect/Triggered Subsystem1 ==
  In1 : Inport
  Trigger : TriggerPort  TriggerType=falling
  Out1 : Outport
  wires:
  In1/1 -> Out1/1

== system FullSystem_threshold_fix_attempt/Decoder /Geortzel Filtering /Frequency Detect 3 /Triggered Subsystem ==
  In1 : Inport
  Trigger : TriggerPort
  Out1 : Outport
  wires:
  In1/1 -> Out1/1

== system FullSystem_threshold_fix_attempt/Decoder /Geortzel Filtering /Frequency Detect 3 /Triggered Subsystem1 ==
  In1 : Inport
  Trigger : TriggerPort  TriggerType=falling
  Out1 : Outport
  wires:
  In1/1 -> Out1/1

== system FullSystem_threshold_fix_attempt/Decoder /Geortzel Filtering /Frequency Detect 4/Triggered Subsystem ==
  In1 : Inport
  Trigger : TriggerPort
  Out1 : Outport
  wires:
  In1/1 -> Out1/1

== system FullSystem_threshold_fix_attempt/Decoder /Geortzel Filtering /Frequency Detect 4/Triggered Subsystem1 ==
  In1 : Inport
  Trigger : TriggerPort  TriggerType=falling
  Out1 : Outport
  wires:
  In1/1 -> Out1/1

== system FullSystem_threshold_fix_attempt/Decoder /Geortzel Filtering /Frequency Detect 6 /Triggered Subsystem ==
  In1 : Inport
  Trigger : TriggerPort
  Out1 : Outport
  wires:
  In1/1 -> Out1/1

== system FullSystem_threshold_fix_attempt/Decoder /Geortzel Filtering /Frequency Detect 6 /Triggered Subsystem1 ==
  In1 : Inport
  Trigger : TriggerPort  TriggerType=falling
  Out1 : Outport
  wires:
  In1/1 -> Out1/1

== system FullSystem_threshold_fix_attempt/Decoder /Geortzel Filtering /Frequency Detect 7 /Triggered Subsystem ==
  In1 : Inport
  Trigger : TriggerPort
  Out1 : Outport
  wires:
  In1/1 -> Out1/1

== system FullSystem_threshold_fix_attempt/Decoder /Geortzel Filtering /Frequency Detect 7 /Triggered Subsystem1 ==
  In1 : Inport
  Trigger : TriggerPort  TriggerType=falling
  Out1 : Outport
  wires:
  In1/1 -> Out1/1

== system FullSystem_threshold_fix_attempt/Decoder /Geortzel Filtering /Frequency Detect1 /Triggered Subsystem ==
  In1 : Inport
  Trigger : TriggerPort
  Out1 : Outport
  wires:
  In1/1 -> Out1/1

== system FullSystem_threshold_fix_attempt/Decoder /Geortzel Filtering /Frequency Detect1 /Triggered Subsystem1 ==
  In1 : Inport
  Trigger : TriggerPort  TriggerType=falling
  Out1 : Outport
  wires:
  In1/1 -> Out1/1

== system FullSystem_threshold_fix_attempt/Decoder /Geortzel Filtering /Frequency Detect2 /Triggered Subsystem ==
  In1 : Inport
  Trigger : TriggerPort
  Out1 : Outport
  wires:
  In1/1 -> Out1/1

== system FullSystem_threshold_fix_attempt/Decoder /Geortzel Filtering /Frequency Detect2 /Triggered Subsystem1 ==
  In1 : Inport
  Trigger : TriggerPort  TriggerType=falling
  Out1 : Outport
  wires:
  In1/1 -> Out1/1

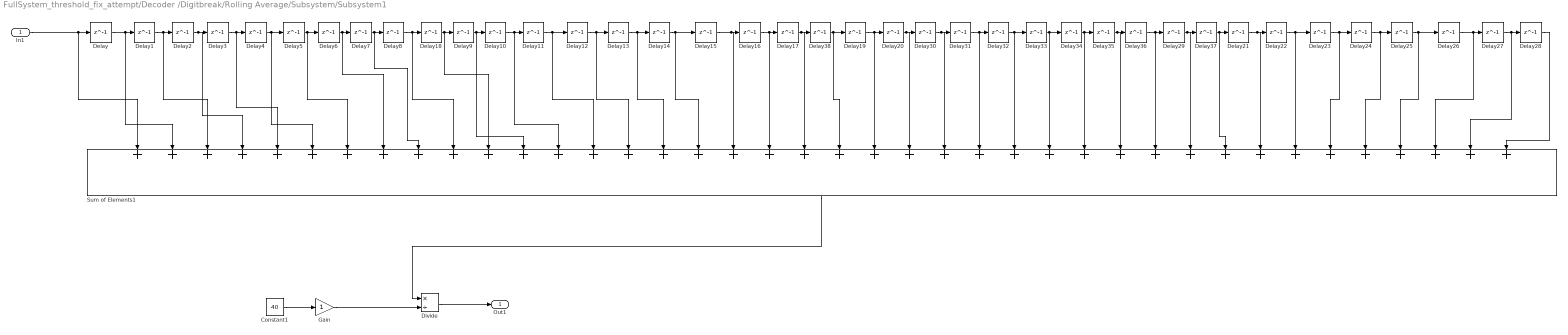
== system FullSystem_threshold_fix_attempt/Decoder /Digitbreak/Rolling Average/Subsystem/Subsystem1 ==
  In1 : Inport
  Constant1 : Constant  Value=40
  Delay{,1..38} (39 alike) : Delay  DelayLength=1  InitialCondition=0
  Divide : Product  Inputs=*/
  Gain : Gain
  Sum of Elements1 : Sum  Inputs=++++++++++++++++++++++++++++++++++++++++
  Out1 : Outport
  wires:
  In1/1 -> Sum of Elements1/1, Delay/1
  Divide/1 -> Out1/1
  Delay2/1 -> Sum of Elements1/4, Delay3/1
  Delay5/1 -> Delay6/1, Sum of Elements1/7
  Delay6/1 -> Delay7/1, Sum of Elements1/8
  Delay7/1 -> Sum of Elements1/9, Delay8/1
  Sum of Elements1/1 -> Divide/1
  Delay4/1 -> Delay5/1, Sum of Elements1/6
  Gain/1 -> Divide/2
  Delay3/1 -> Delay4/1, Sum of Elements1/5
  Delay1/1 -> Sum of Elements1/3, Delay2/1
  Constant1/1 -> Gain/1
  Delay/1 -> Sum of Elements1/2, Delay1/1
  Delay8/1 -> Delay18/1, Sum of Elements1/10
  Delay11/1 -> Sum of Elements1/14, Delay12/1
  Delay14/1 -> Sum of Elements1/17, Delay15/1
  Delay15/1 -> Sum of Elements1/18, Delay16/1
  Delay16/1 -> Sum of Elements1/19, Delay17/1
  Delay17/1 -> Sum of Elements1/20, Delay38/1
  Delay13/1 -> Sum of Elements1/16, Delay14/1
  Delay12/1 -> Sum of Elements1/15, Delay13/1
  Delay10/1 -> Sum of Elements1/13, Delay11/1
  Delay9/1 -> Sum of Elements1/12, Delay10/1
  Delay18/1 -> Sum of Elements1/11, Delay9/1
  Delay30/1 -> Sum of Elements1/24, Delay31/1
  Delay33/1 -> Sum of Elements1/27, Delay34/1
  Delay34/1 -> Sum of Elements1/28, Delay35/1
  Delay35/1 -> Sum of Elements1/29, Delay36/1
  Delay32/1 -> Sum of Elements1/26, Delay33/1
  Delay31/1 -> Sum of Elements1/25, Delay32/1
  Delay20/1 -> Sum of Elements1/23, Delay30/1
  Delay36/1 -> Sum of Elements1/30, Delay29/1
  Delay22/1 -> Sum of Elements1/34, Delay23/1
  Delay25/1 -> Sum of Elements1/37, Delay26/1
  Delay26/1 -> Sum of Elements1/38, Delay27/1
  Delay27/1 -> Sum of Elements1/39, Delay28/1
  Delay28/1 -> Sum of Elements1/40
  Delay24/1 -> Sum of Elements1/36, Delay25/1
  Delay23/1 -> Sum of Elements1/35, Delay24/1
  Delay21/1 -> Sum of Elements1/33, Delay22/1
  Delay37/1 -> Sum of Elements1/32, Delay21/1
  Delay29/1 -> Sum of Elements1/31, Delay37/1
  Delay38/1 -> Delay19/1, Sum of Elements1/21
  Delay19/1 -> Sum of Elements1/22, Delay20/1
